simulink model "Model_02_Rotor_Reference_Frame_Transformation"  (R2020a)
settings: Solver=ode4  StartTime=0.0  StopTime=2  FixedStep=1e-4  RelTol=1e-3
settings Model: Creator=samee  LastModifiedBy=DEVIKAT
settings DebuggingCC: UnconnectedInputMsg=none  UnconnectedOutputMsg=none  UnconnectedLineMsg=none

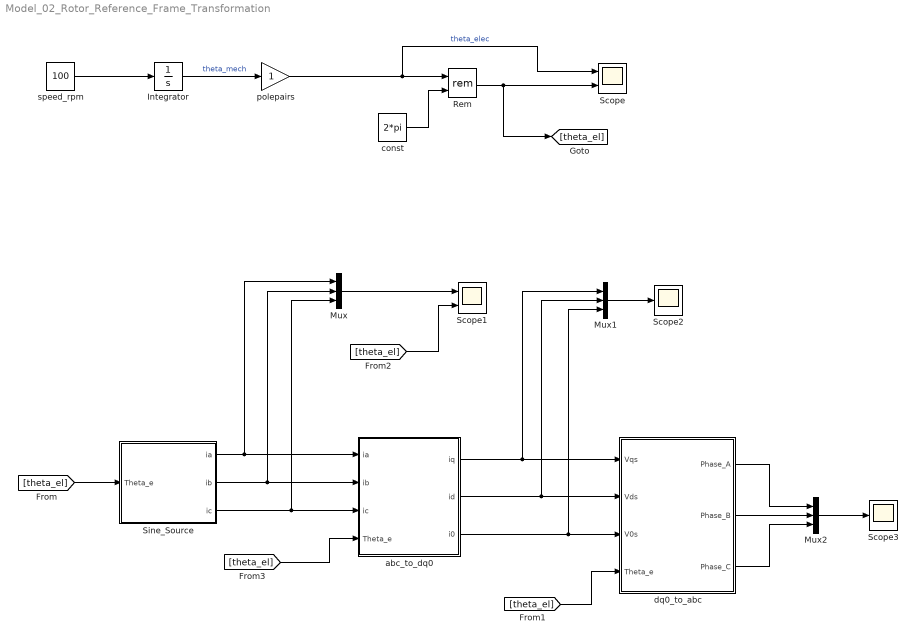
== system Model_02_Rotor_Reference_Frame_Transformation ==
  Integrator : Integrator
  Mux : Mux  Inputs=3
  Mux1 : Mux  Inputs=3
  Mux2 : Mux  Inputs=3
  Rem : Math  Operator=rem  SaturateOnIntegerOverflow=on
  Scope : Scope  NumInputPorts=2
  Scope1 : Scope  NumInputPorts=2
  Scope2 : Scope
  Scope3 : Scope
  Sine_Source : MATLAB Function  TreatAsAtomicUnit=on
  abc_to_dq0 : MATLAB Function  TreatAsAtomicUnit=on
  const : Constant  Value=2*pi
  dq0_to_abc : MATLAB Function  TreatAsAtomicUnit=on
  polepairs : Gain
  speed_rpm : Constant  Value=100
  wires:
  Integrator/1 -> polepairs/1  "theta_mech"
  polepairs/1 -> Scope/1, Rem/1  "theta_elec"
  const/1 -> Rem/2
  Rem/1 -> [theta_el], Scope/2
  speed_rpm/1 -> Integrator/1
  [theta_el] -> Sine_Source/1(Theta_e)
  Sine_Source/1(ia) -> Mux/1, abc_to_dq0/1(ia)
  Sine_Source/2(ib) -> Mux/2, abc_to_dq0/2(ib)
  Sine_Source/3(ic) -> Mux/3, abc_to_dq0/3(ic)
  abc_to_dq0/1(iq) -> dq0_to_abc/1(Vqs), Mux1/1
  abc_to_dq0/2(id) -> Mux1/2, dq0_to_abc/2(Vds)
  abc_to_dq0/3(i0) -> Mux1/3, dq0_to_abc/3(V0s)
  [theta_el] -> dq0_to_abc/4(Theta_e)
  Mux/1 -> Scope1/1
  [theta_el] -> Scope1/2
  [theta_el] -> abc_to_dq0/4(Theta_e)
  Mux1/1 -> Scope2/1
  dq0_to_abc/1(Phase_A) -> Mux2/1
  dq0_to_abc/2(Phase_B) -> Mux2/2
  dq0_to_abc/3(Phase_C) -> Mux2/3
  Mux2/1 -> Scope3/1

== matlab function Model_02_Rotor_Reference_Frame_Transformation/abc_to_dq0 ==
  data: ia input; iq output; ib input; ic input; Theta_e input; id output; i0 output
function [iq, id, i0] = fcn(ia, ib, ic, Theta_e)
%#codegen
% Ks    =   (2/3)*[ cos(Theta_e)        cos(Theta_e-(2*pi/3))           cos(Theta_e+(2*pi/3));
%                   sin (Theta_e)       sin (Theta_e-(2*pi/3))          sin(Theta_e+(2*pi/3));
%                   0.5                 0.5                             0.5 ];
% 
% iqd0  =   Ks*[ia;ib;ic];
% 
% iq    =   iqd0(1);
% id    =   iqd0(2);
% 10    =   iqd0(3);

iq = (2/3)*(cos(Theta_e)*ia + cos(Theta_e-(2*pi/3))*ib + cos(Theta_e+(2*pi/3))*ic); 
id = (2/3)*(sin(Theta_e)*ia + sin(Theta_e-(2*pi/3))*ib + sin(Theta_e+(2*pi/3))*ic); 
i0 = (2/3)*(0.5*ia + 0.5*ib + 0.5*ic);

== matlab function Model_02_Rotor_Reference_Frame_Transformation/dq0_to_abc ==
  data: Vqs input; Phase_A output; Vds input; V0s input; Theta_e input; Phase_B output; Phase_C output
function [Phase_A, Phase_B, Phase_C] = fcn(Vqs, Vds, V0s, Theta_e)
%#codegen

% if Time < 1
%     Phase_U = Amplitude*sin(Theta);
%     Phase V = Amplitude*sin(Theta-2*pi/3);
%     Phase_W = Amplitude*sin(Theta-4*pi/3);
% else
%     Phase_U = Amplitude*sin(Theta + (pi/18));
%     Phase V = Amplitude*sin(Theta - 2*pi/3 + (pi/18));
%     Phase W = Amplitude*sin(Theta - 4*pi/3 + (pi/18));
% end
%     Phase_U = Amplitude*cos(Theta);
%     Phase_V = Amplitude*cos(Theta-(2*pi/3));
%     Phase W = Amplitude*cos(Theta-(4*pi/3));
%
%
%
% Phase Advance
% Theta = Theta_e+ (p1/30);
Theta = Theta_e + (0);

Phase_A = cos(Theta)*Vqs + sin(Theta)*Vds + V0s*1;
Phase_B = cos(Theta-(2*pi/3))*Vqs + sin(Theta - (2*pi/3))*Vds + V0s*1;
Phase_C = cos(Theta+(2*pi/3))*Vqs + sin(Theta + (2*pi/3))*Vds + V0s*1;

== matlab function Model_02_Rotor_Reference_Frame_Transformation/Sine_Source ==
  data: ia output; Theta_e input; ib output; ic output
function [ia,ib, ic] = fcn(Theta_e)
%#codegen

ia = 1*cos(Theta_e);
ib = 1*cos(Theta_e - (2*pi/3));
ic = cos(Theta_e + (2*pi/3));
